simulink model "Quad_Cascade_PID"  (R2021b)
settings: Solver=ode45  StartTime=0.0  StopTime=t_sim  MaxStep=0.01  RelTol=1e-3  AbsTol=1e-6
values from neighbouring files (symbols this model uses):
  att_cmd_limit = 18 * pi/180    (= 0.314159265359)    [Quad_Params.m]
  AW_Phi = 0.5    [Quad_Params.m]
  AW_Psi = 0.3    [Quad_Params.m]
  AW_Theta = 0.5    [Quad_Params.m]
  AW_X = 0.5    [Quad_Params.m]
  AW_Y = 0.5    [Quad_Params.m]
  AW_Z = 3.0    (= 3)    [Quad_Params.m]
  B_torque = 0.0382    [Quad_Params.m]
  FF_X = 0.35    [Quad_Params.m]
  FF_Y = 0.40    (= 0.4)    [Quad_Params.m]
  g = 9.81    [Quad_Params.m]
  IXX = 4.856e-3    (= 0.004856)    [Quad_Params.m]
  IYY = 4.856e-3    (= 0.004856)    [Quad_Params.m]
  IZZ = 8.801e-3    (= 0.008801)    [Quad_Params.m]
  K_thrust = 2.98e-6    (= 2.98e-06)    [Quad_Params.m]
  KD_P = 0.010    (= 0.01)    [Quad_Params.m]
  KD_Phi = 0.80    (= 0.8)    [Quad_Params.m]
  KD_Psi = 0.40    (= 0.4)    [Quad_Params.m]
  KD_Q = 0.010    (= 0.01)    [Quad_Params.m]
  KD_R = 0.008    [Quad_Params.m]
  KD_Theta = 0.80    (= 0.8)    [Quad_Params.m]
  KD_X = 0.50    (= 0.5)    [Quad_Params.m]
  KD_Y = 0.70    (= 0.7)    [Quad_Params.m]
  KD_Z = 1.50    (= 1.5)    [Quad_Params.m]
  KI_P = 0.0001    [Quad_Params.m]
  KI_Phi = 0.0001    [Quad_Params.m]
  KI_Psi = 0.5    [Quad_Params.m]
  KI_Q = 0.0001    [Quad_Params.m]
  KI_R = 0.0001    [Quad_Params.m]
  KI_Theta = 0.0001    [Quad_Params.m]
  KI_X = 0.00    (= 0)    [Quad_Params.m]
  KI_Y = 0.00    (= 0)    [Quad_Params.m]
  KI_Z = 10.0    (= 10)    [Quad_Params.m]
  KP_P = 0.80    (= 0.8)    [Quad_Params.m]
  KP_Phi = 6.0    (= 6)    [Quad_Params.m]
  KP_Psi = 4.0    (= 4)    [Quad_Params.m]
  KP_Q = 0.80    (= 0.8)    [Quad_Params.m]
  KP_R = 0.60    (= 0.6)    [Quad_Params.m]
  KP_Theta = 6.0    (= 6)    [Quad_Params.m]
  KP_X = 0.80    (= 0.8)    [Quad_Params.m]
  KP_Y = 1.00    (= 1)    [Quad_Params.m]
  KP_Z = 10.0    (= 10)    [Quad_Params.m]
  L = 0.225    [Quad_Params.m]
  m = 0.468    [Quad_Params.m]    (also in quad_plant_fcn.m)
  M_max = L * K_thrust * omega_max^2    (= 0.6705)    [Quad_Params.m]
  N_rate = 50    [Quad_Params.m]
  omega_sq_max = omega_max^2    (= 1000000)    [Quad_Params.m]
  omega_sq_min = 0    [Quad_Params.m]
  Psid = 0.0    (= 0)    [Quad_Params.m]
  T_max = 4 * K_thrust * omega_max^2    (= 11.92)    [Quad_Params.m]
  T_min = 0    [Quad_Params.m]
  Ts_inner = 0.005    [Quad_Params.m]
  Ts_mid = 0.010    (= 0.01)    [Quad_Params.m]
  Ts_outer = 0.020    (= 0.02)    [Quad_Params.m]
  yaw_rate_limit = 1.0    (= 1)    [Quad_Params.m]
settings Model: Creator=ADMIN  LastModifiedBy=ADMIN
settings DataIOCC: SaveFormat=Array  ReturnWorkspaceOutputs=off

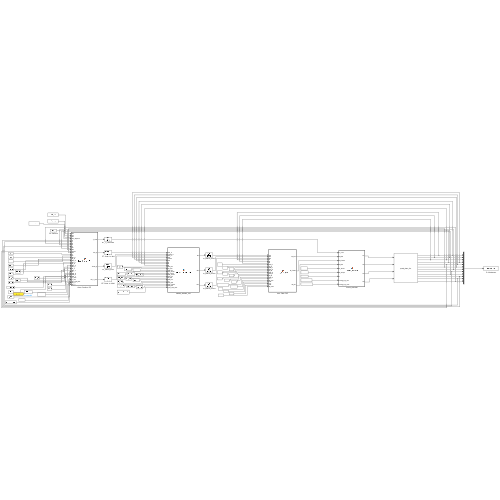
[thumbnail: Simulink's stored preview of the top-level diagram]
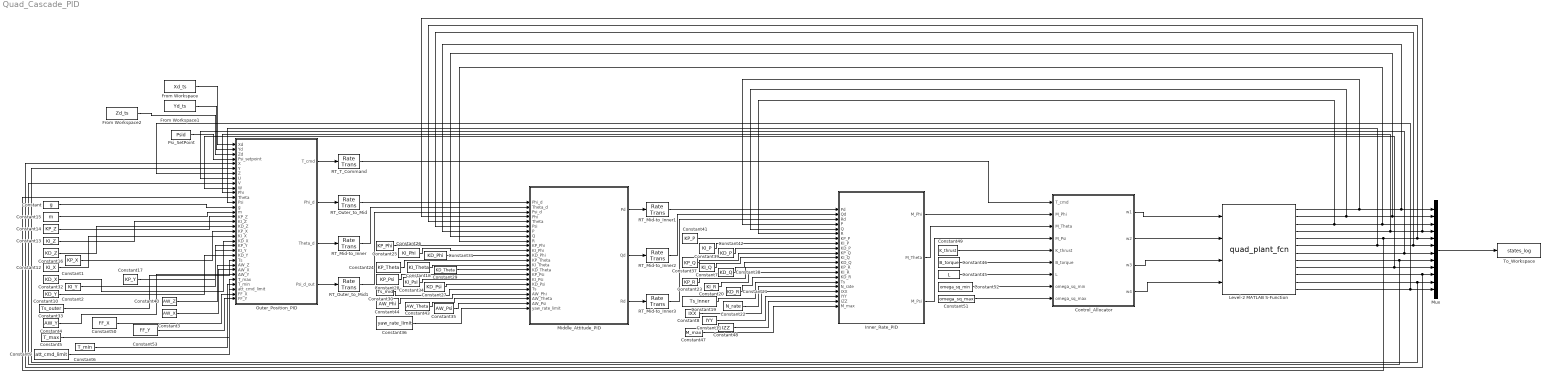
== system Quad_Cascade_PID ==
  Constant : Constant  Value=g
  Constant1 : Constant  Value=KP_X
  Constant10 : Constant  Value=KD_Y
  Constant11 : Constant  Value=IYY
  Constant12 : Constant  Value=KI_X
  Constant13 : Constant  Value=KI_Z
  Constant14 : Constant  Value=KP_Z
  Constant15 : Constant  Value=m
  Constant16 : Constant  Value=KD_Z
  Constant17 : Constant  Value=KP_Y
  Constant18 : Constant  Value=KI_Theta
  Constant19 : Constant  Value=Ts_inner
  Constant2 : Constant  Value=KI_Y
  Constant20 : Constant  Value=KI_R
  Constant21 : Constant  Value=KD_R
  Constant22 : Constant  Value=N_rate
  Constant23 : Constant  Value=KP_R
  Constant24 : Constant  Value=KP_Theta
  Constant25 : Constant  Value=KP_Phi
  Constant26 : Constant  Value=KI_Phi
  Constant27 : Constant  Value=KD_Psi
  Constant28 : Constant  Value=KP_Psi
  Constant29 : Constant  Value=KD_Theta
  Constant3 : Constant  Value=AW_X
  Constant30 : Constant  Value=Ts_mid
  Constant31 : Constant  Value=KD_Phi
  Constant32 : Constant  Value=KD_X
  Constant33 : Constant  Value=Ts_outer
  Constant34 : Constant  Value=KI_Psi
  Constant35 : Constant  Value=AW_Psi
  Constant36 : Constant  Value=yaw_rate_limit
  Constant37 : Constant  Value=KP_Q
  Constant38 : Constant  Value=KD_Q
  Constant39 : Constant  Value=KI_P
  Constant4 : Constant  Value=AW_Y
  Constant40 : Constant  Value=AW_Z
  Constant41 : Constant  Value=KP_P
  Constant42 : Constant  Value=KD_P
  Constant43 : Constant  Value=AW_Theta
  Constant44 : Constant  Value=AW_Phi
  Constant45 : Constant  Value=L
  Constant46 : Constant  Value=B_torque
  Constant47 : Constant  Value=M_max
  Constant48 : Constant  Value=IZZ
  Constant49 : Constant  Value=K_thrust
  Constant5 : Constant  Value=T_max
  Constant50 : Constant  Value=FF_X
  Constant51 : Constant  Value=omega_sq_max
  Constant52 : Constant  Value=omega_sq_min
  Constant53 : Constant  Value=FF_Y
  Constant6 : Constant  Value=T_min
  Constant7 : Constant  Value=KI_Q
  Constant8 : Constant  Value=IXX
  Constant9 : Constant  Value=att_cmd_limit
  Control_Allocator : MATLAB Function  TreatAsAtomicUnit=on
  From Workspace : FromWorkspace  VariableName=Xd_ts
  From Workspace1 : FromWorkspace  VariableName=Yd_ts
  From Workspace2 : FromWorkspace  VariableName=Zd_ts
  Inner_Rate_PID : MATLAB Function  TreatAsAtomicUnit=on  SystemSampleTime=Ts_inner
  Level-2 MATLAB S-Function : M-S-Function  FunctionName=quad_plant_fcn
  Middle_Attitude_PID : MATLAB Function  TreatAsAtomicUnit=on  SystemSampleTime=Ts_mid
  Mux : Mux  Inputs=12
  Outer_Position_PID : MATLAB Function  TreatAsAtomicUnit=on  SystemSampleTime=Ts_outer
  Psi_SetPoint : Constant  Value=Psid
  RT_Mid-to_Inner{,1..3} (4 alike) : RateTransition  Deterministic=off  OutPortSampleTime=Ts_inner
  RT_Outer_to_Mid : RateTransition  Deterministic=off  OutPortSampleTime=Ts_inner
  RT_Outer_to_Mid1 : RateTransition  Deterministic=off  OutPortSampleTime=Ts_inner
  RT_T_Command : RateTransition  Deterministic=off  OutPortSampleTime=Ts_inner
  To_Workspace : ToWorkspace  VariableName=states_log  SampleTime=-1
  wires:
  Level-2 MATLAB S-Function/1 -> Inner_Rate_PID/4(P), Middle_Attitude_PID/7(P), Mux/1
  Level-2 MATLAB S-Function/2 -> Inner_Rate_PID/5(Q), Middle_Attitude_PID/8(Q), Mux/2
  Level-2 MATLAB S-Function/3 -> Inner_Rate_PID/6(R), Middle_Attitude_PID/9(R), Mux/3
  Level-2 MATLAB S-Function/4 -> Middle_Attitude_PID/4(Phi), Mux/4, Outer_Position_PID/11(Phi)
  Level-2 MATLAB S-Function/5 -> Middle_Attitude_PID/5(Theta), Mux/5, Outer_Position_PID/12(Theta)
  Level-2 MATLAB S-Function/6 -> Middle_Attitude_PID/6(Psi), Mux/6, Outer_Position_PID/13(Psi)
  Level-2 MATLAB S-Function/7 -> Outer_Position_PID/8(U), Mux/7
  Level-2 MATLAB S-Function/8 -> Outer_Position_PID/9(V), Mux/8
  Level-2 MATLAB S-Function/9 -> Outer_Position_PID/10(W), Mux/9
  Level-2 MATLAB S-Function/10 -> Outer_Position_PID/5(X), Mux/10
  Level-2 MATLAB S-Function/11 -> Outer_Position_PID/6(Y), Mux/11
  Level-2 MATLAB S-Function/12 -> Outer_Position_PID/7(Z), Mux/12
  Mux/1 -> To_Workspace/1
  Psi_SetPoint/1 -> Outer_Position_PID/4(Psi_setpoint)
  Constant9/1 -> Outer_Position_PID/31(att_cmd_limit)
  Constant6/1 -> Outer_Position_PID/30(T_min)
  Constant5/1 -> Outer_Position_PID/29(T_max)
  Constant4/1 -> Outer_Position_PID/28(AW_Y)
  Constant3/1 -> Outer_Position_PID/27(AW_X)
  Constant40/1 -> Outer_Position_PID/26(AW_Z)
  Constant33/1 -> Outer_Position_PID/25(Ts)
  Constant10/1 -> Outer_Position_PID/24(KD_Y)
  Constant2/1 -> Outer_Position_PID/23(KI_Y)
  Constant17/1 -> Outer_Position_PID/22(KP_Y)
  Constant32/1 -> Outer_Position_PID/21(KD_X)
  Constant12/1 -> Outer_Position_PID/20(KI_X)
  Constant1/1 -> Outer_Position_PID/19(KP_X)
  Constant16/1 -> Outer_Position_PID/18(KD_Z)
  Constant13/1 -> Outer_Position_PID/17(KI_Z)
  Constant14/1 -> Outer_Position_PID/16(KP_Z)
  Constant15/1 -> Outer_Position_PID/15(m)
  Constant/1 -> Outer_Position_PID/14(g)
  Outer_Position_PID/1(T_cmd) -> RT_T_Command/1
  Outer_Position_PID/2(Phi_d) -> RT_Outer_to_Mid/1
  Outer_Position_PID/3(Theta_d) -> RT_Mid-to_Inner/1
  Outer_Position_PID/4(Psi_d_out) -> RT_Outer_to_Mid1/1
  RT_Outer_to_Mid/1 -> Middle_Attitude_PID/1(Phi_d)
  RT_Mid-to_Inner/1 -> Middle_Attitude_PID/2(Theta_d)
  RT_Outer_to_Mid1/1 -> Middle_Attitude_PID/3(Psi_d)
  Constant25/1 -> Middle_Attitude_PID/10(KP_Phi)
  Constant26/1 -> Middle_Attitude_PID/11(KI_Phi)
  Constant31/1 -> Middle_Attitude_PID/12(KD_Phi)
  Constant24/1 -> Middle_Attitude_PID/13(KP_Theta)
  Constant18/1 -> Middle_Attitude_PID/14(KI_Theta)
  Constant29/1 -> Middle_Attitude_PID/15(KD_Theta)
  Constant28/1 -> Middle_Attitude_PID/16(KP_Psi)
  Constant34/1 -> Middle_Attitude_PID/17(KI_Psi)
  Constant27/1 -> Middle_Attitude_PID/18(KD_Psi)
  Constant30/1 -> Middle_Attitude_PID/19(Ts)
  Constant44/1 -> Middle_Attitude_PID/20(AW_Phi)
  Constant43/1 -> Middle_Attitude_PID/21(AW_Theta)
  Constant35/1 -> Middle_Attitude_PID/22(AW_Psi)
  Constant36/1 -> Middle_Attitude_PID/23(yaw_rate_limit)
  Middle_Attitude_PID/1(Pd) -> RT_Mid-to_Inner1/1
  Middle_Attitude_PID/2(Qd) -> RT_Mid-to_Inner2/1
  Middle_Attitude_PID/3(Rd) -> RT_Mid-to_Inner3/1
  RT_Mid-to_Inner1/1 -> Inner_Rate_PID/1(Pd)
  RT_Mid-to_Inner2/1 -> Inner_Rate_PID/2(Qd)
  RT_Mid-to_Inner3/1 -> Inner_Rate_PID/3(Rd)
  Constant41/1 -> Inner_Rate_PID/7(KP_P)
  Constant39/1 -> Inner_Rate_PID/8(KI_P)
  Constant42/1 -> Inner_Rate_PID/9(KD_P)
  Constant37/1 -> Inner_Rate_PID/10(KP_Q)
  Constant7/1 -> Inner_Rate_PID/11(KI_Q)
  Constant38/1 -> Inner_Rate_PID/12(KD_Q)
  Constant23/1 -> Inner_Rate_PID/13(KP_R)
  Constant20/1 -> Inner_Rate_PID/14(KI_R)
  Constant21/1 -> Inner_Rate_PID/15(KD_R)
  Constant19/1 -> Inner_Rate_PID/16(Ts)
  Constant22/1 -> Inner_Rate_PID/17(N_rate)
  Constant8/1 -> Inner_Rate_PID/18(IXX)
  Constant11/1 -> Inner_Rate_PID/19(IYY)
  Constant48/1 -> Inner_Rate_PID/20(IZZ)
  Constant47/1 -> Inner_Rate_PID/21(M_max)
  Inner_Rate_PID/1(M_Phi) -> Control_Allocator/2(M_Phi)
  Inner_Rate_PID/2(M_Theta) -> Control_Allocator/3(M_Theta)
  Inner_Rate_PID/3(M_Psi) -> Control_Allocator/4(M_Psi)
  RT_T_Command/1 -> Control_Allocator/1(T_cmd)
  Constant49/1 -> Control_Allocator/5(K_thrust)
  Constant46/1 -> Control_Allocator/6(B_torque)
  Constant45/1 -> Control_Allocator/7(L)
  Constant52/1 -> Control_Allocator/8(omega_sq_min)
  Constant51/1 -> Control_Allocator/9(omega_sq_max)
  Control_Allocator/1(w1) -> Level-2 MATLAB S-Function/1
  Control_Allocator/2(w2) -> Level-2 MATLAB S-Function/2
  Control_Allocator/3(w3) -> Level-2 MATLAB S-Function/3
  Control_Allocator/4(w4) -> Level-2 MATLAB S-Function/4
  From Workspace2/1 -> Outer_Position_PID/3(Zd)
  From Workspace1/1 -> Outer_Position_PID/2(Yd)
  From Workspace/1 -> Outer_Position_PID/1(Xd)
  Constant50/1 -> Outer_Position_PID/32(FF_X)
  Constant53/1 -> Outer_Position_PID/33(FF_Y)

== matlab function Quad_Cascade_PID/Inner_Rate_PID ==
  data: Pd input; M_Phi output; Qd input; Rd input; P input; Q input; R input; M_Theta output; M_Psi output; KP_P input; KI_P input; KD_P input; KP_Q input; KI_Q input; KD_Q input; KP_R input; KI_R input; KD_R input; Ts input; N_rate input; IXX input; IYY input; IZZ input; M_max input
function [M_Phi, M_Theta, M_Psi] = Inner_Rate_PID(...
    Pd, Qd, Rd, P, Q, R, ...
    KP_P, KI_P, KD_P, ...
    KP_Q, KI_Q, KD_Q, ...
    KP_R, KI_R, KD_R, ...
    Ts, N_rate, ...
    IXX, IYY, IZZ, M_max)

% INNER RATE PID
% All parameters passed directly as input ports

% Persistent states
persistent int_P int_Q int_R prev_eP prev_eQ prev_eR first_run

if isempty(first_run)
    int_P    = 0;   int_Q    = 0;   int_R    = 0;
    prev_eP  = 0;   prev_eQ  = 0;   prev_eR  = 0;
    first_run = false;
end

% =============================================
% RATE ERRORS
% =============================================

eP = Pd - P;
eQ = Qd - Q;
eR = Rd - R;

% =============================================
% INTEGRATOR UPDATE (Tustin)
% =============================================

int_P = int_P + (Ts/2) * (eP + prev_eP);
int_Q = int_Q + (Ts/2) * (eQ + prev_eQ);
int_R = int_R + (Ts/2) * (eR + prev_eR);

% =============================================
% DERIVATIVE WITH FILTER
% =============================================

dP = N_rate * (eP - prev_eP) / (1 + N_rate * Ts);
dQ = N_rate * (eQ - prev_eQ) / (1 + N_rate * Ts);
dR = N_rate * (eR - prev_eR) / (1 + N_rate * Ts);

% =============================================
% PID OUTPUT — torque commands
% Multiply by inertia for physical units [N.m]
% =============================================

M_Phi_raw   = IXX * (KP_P * eP + KI_P * int_P + KD_P * dP);
M_Theta_raw = IYY * (KP_Q * eQ + KI_Q * int_Q + KD_Q * dQ);
M_Psi_raw   = IZZ * (KP_R * eR + KI_R * int_R + KD_R * dR);

% Saturate torques
M_Phi   = max(-M_max, min(M_max, M_Phi_raw));
M_Theta = max(-M_max, min(M_max, M_Theta_raw));
M_Psi   = max(-M_max, min(M_max, M_Psi_raw));

% Back-calculation anti-windup
AW_gain = 0.1;
int_P = int_P + AW_gain * (M_Phi   - M_Phi_raw)   / (IXX * KI_P + eps);
int_Q = int_Q + AW_gain * (M_Theta - M_Theta_raw) / (IYY * KI_Q + eps);
int_R = int_R + AW_gain * (M_Psi   - M_Psi_raw)   / (IZZ * KI_R + eps);

% =============================================
% UPDATE MEMORY
% =============================================

prev_eP = eP;
prev_eQ = eQ;
prev_eR = eR;

end

== matlab function Quad_Cascade_PID/Control_Allocator ==
  data: T_cmd input; w1 output; M_Phi input; M_Theta input; M_Psi input; w2 output; w3 output; w4 output; K_thrust input; B_torque input; L input; omega_sq_min input; omega_sq_max input
function [w1, w2, w3, w4] = Control_Allocator(...
    T_cmd, M_Phi, M_Theta, M_Psi, ...
    K_thrust, B_torque, L, ...
    omega_sq_min, omega_sq_max)

% CONTROL ALLOCATOR
% All parameters passed directly as input ports

% =============================================
% STEP 1: Compute omega squared (Eq. 3.24)
% =============================================

T_over_4K      = T_cmd    / (4 * K_thrust);
M_theta_term   = M_Theta  / (2 * K_thrust * L);
M_phi_term     = M_Phi    / (2 * K_thrust * L);
M_psi_term     = M_Psi    / (4 * B_torque);

w1_sq = T_over_4K - M_theta_term - M_psi_term;
w2_sq = T_over_4K - M_phi_term   + M_psi_term;
w3_sq = T_over_4K + M_theta_term - M_psi_term;
w4_sq = T_over_4K + M_phi_term   + M_psi_term;

% =============================================
% STEP 2: Physical saturation
% omega squared cannot be negative
% =============================================

w1_sq = max(omega_sq_min, min(omega_sq_max, w1_sq));
w2_sq = max(omega_sq_min, min(omega_sq_max, w2_sq));
w3_sq = max(omega_sq_min, min(omega_sq_max, w3_sq));
w4_sq = max(omega_sq_min, min(omega_sq_max, w4_sq));

% =============================================
% STEP 3: Square root to get rotor speeds
% =============================================

w1 = sqrt(w1_sq);
w2 = sqrt(w2_sq);
w3 = sqrt(w3_sq);
w4 = sqrt(w4_sq);

end

== matlab function Quad_Cascade_PID/Middle_Attitude_PID ==
  data: Phi_d input; Pd output; Theta_d input; Psi_d input; Phi input; Theta input; Psi input; P input; Q input; R input; Qd output; Rd output; KP_Phi input; KI_Phi input; KD_Phi input; KP_Theta input; KI_Theta input; KD_Theta input; KP_Psi input; KI_Psi input; KD_Psi input; Ts input; AW_Phi input; AW_Theta input; AW_Psi input; yaw_rate_limit input
function [Pd, Qd, Rd] = Middle_Attitude_PID(...
    Phi_d, Theta_d, Psi_d, ...
    Phi, Theta, Psi, P, Q, R, ...
    KP_Phi, KI_Phi, KD_Phi, ...
    KP_Theta, KI_Theta, KD_Theta, ...
    KP_Psi, KI_Psi, KD_Psi, ...
    Ts, AW_Phi, AW_Theta, AW_Psi, ...
    yaw_rate_limit)

% MIDDLE ATTITUDE PID
% All parameters passed directly as input ports

% Persistent integrator states
persistent int_Phi int_Theta int_Psi first_run

if isempty(first_run)
    int_Phi   = 0;
    int_Theta = 0;
    int_Psi   = 0;
    first_run = false;
end

% =============================================
% ANGLE ERRORS
% =============================================

e_Phi   = Phi_d   - Phi;
e_Theta = Theta_d - Theta;

% Wrap yaw error to [-pi, pi]
e_Psi_raw = Psi_d - Psi;
e_Psi     = atan2(sin(e_Psi_raw), cos(e_Psi_raw));

% =============================================
% INTEGRATOR UPDATE
% =============================================

int_Phi   = int_Phi   + Ts * e_Phi;
int_Theta = int_Theta + Ts * e_Theta;
int_Psi   = int_Psi   + Ts * e_Psi;

% Anti-windup clamping
int_Phi   = max(-AW_Phi/KI_Phi,     min(AW_Phi/KI_Phi,     int_Phi));
int_Theta = max(-AW_Theta/KI_Theta, min(AW_Theta/KI_Theta, int_Theta));
int_Psi   = max(-AW_Psi/KI_Psi,     min(AW_Psi/KI_Psi,     int_Psi));

% =============================================
% DERIVATIVE ON MEASUREMENT
% Uses actual rates P, Q, R instead of
% differentiating error — no derivative kick
% =============================================

dPhi_meas   = -P;
dTheta_meas = -Q;
dPsi_meas   = -R;

% =============================================
% PID OUTPUT — desired angular rates
% =============================================

rate_lim = yaw_rate_limit * 3;

Pd_raw = KP_Phi   * e_Phi   + KI_Phi   * int_Phi   + KD_Phi   * dPhi_meas;
Qd_raw = KP_Theta * e_Theta + KI_Theta * int_Theta + KD_Theta * dTheta_meas;
Rd_raw = KP_Psi   * e_Psi   + KI_Psi   * int_Psi   + KD_Psi   * dPsi_meas;

% Saturate output rates
Pd = max(-rate_lim,        min(rate_lim,        Pd_raw));
Qd = max(-rate_lim,        min(rate_lim,        Qd_raw));
Rd = max(-yaw_rate_limit,  min(yaw_rate_limit,  Rd_raw));

end

== matlab function Quad_Cascade_PID/Outer_Position_PID ==
  data: Xd input; T_cmd output; Yd input; Zd input; Psi_setpoint input; X input; Y input; Z input; U input; V input; W input; Phi input; Theta input; Psi input; Phi_d output; Theta_d output; Psi_d_out output; g input; m input; KP_Z input; KI_Z input; KD_Z input; KP_X input; KI_X input; KD_X input; KP_Y input; KI_Y input; KD_Y input; Ts input; AW_Z input; AW_X input; AW_Y input; T_max input; T_min input; att_cmd_limit input; FF_X input; FF_Y input
function [T_cmd, Phi_d, Theta_d, Psi_d_out] = Outer_Position_PID(...
    Xd, Yd, Zd, Psi_setpoint, ...
    X, Y, Z, U, V, W, Phi, Theta, Psi, ...
    g, m, ...
    KP_Z, KI_Z, KD_Z, ...
    KP_X, KI_X, KD_X, ...
    KP_Y, KI_Y, KD_Y, ...
    Ts, AW_Z, AW_X, AW_Y, ...
    T_max, T_min, att_cmd_limit, ...
    FF_X, FF_Y)

% OUTER POSITION PID
% All parameters passed directly as input ports
% FF_X and FF_Y are feedforward gains for X and Y axes

% Persistent integrator states
persistent int_Z int_X int_Y first_run Xd_prev Yd_prev

if isempty(first_run)
    int_Z     = 0;
    int_X     = 0;
    int_Y     = 0;
    Xd_prev   = Xd;
    Yd_prev   = Yd;
    first_run = false;
end

% =============================================
% ALTITUDE CONTROLLER (Z axis)
% =============================================

e_Z = Zd - Z;

% Integrator update
int_Z = int_Z + Ts * e_Z;

% Anti-windup clamping
int_Z = max(-AW_Z, min(AW_Z, int_Z));

% Derivative on measurement
dZ_meas = -W;

% PID output
az_cmd = KP_Z * e_Z + KI_Z * int_Z + KD_Z * dZ_meas;

% Thrust command with gravity feedforward
cos_corr = cos(Phi) * cos(Theta);
cos_corr = max(0.5, cos_corr);
T_raw    = m * (g + az_cmd) / cos_corr;

% Saturate thrust
T_cmd = max(T_min, min(T_max, T_raw));

% =============================================
% HORIZONTAL POSITION CONTROLLER (X, Y)
% =============================================

% Inertial position errors
e_X_inertial = Xd - X;
e_Y_inertial = Yd - Y;

% Rotate to body frame using current yaw
e_X_body =  e_X_inertial * cos(Psi) + e_Y_inertial * sin(Psi);
e_Y_body =  e_Y_inertial * cos(Psi) - e_X_inertial * sin(Psi);

% Desired body velocities
Ud_desired = e_X_body;
Vd_desired = e_Y_body;

% Velocity errors
e_U = Ud_desired - U;
e_V = Vd_desired - V;

% Integrator update with anti-windup
int_X = int_X + Ts * e_U;
int_Y = int_Y + Ts * e_V;
int_X = max(-AW_X, min(AW_X, int_X));
int_Y = max(-AW_Y, min(AW_Y, int_Y));

% Derivative on measurement
dU_meas = -U;
dV_meas = -V;

% =============================================
% FEEDFORWARD CALCULATION
%
% PURPOSE:
%   Normal PID reacts AFTER error builds up.
%   Feedforward predicts where reference is going
%   and acts BEFORE error builds up.
%   This reduces phase lag between lime green and yellow paths.
%
% METHOD:
%   Finite difference of Xd and Yd gives reference velocity.
%   Xd_dot = (Xd_now - Xd_previous) / Ts
%   Yd_dot = (Yd_now - Yd_previous) / Ts
%   Velocity is rotated to body frame using Psi.
%   Then added directly to PID attitude output.
%
% TUNING:
%   FF_X = FF_Y = 0.0  → no feedforward (pure PID)
%   FF_X = FF_Y = 0.5  → medium (current setting)
%   FF_X = FF_Y = 1.0  → strong
%   Cyan lags behind yellow  → increase FF_X, FF_Y
%   Cyan overshoots yellow   → decrease FF_X, FF_Y
% =============================================

% Reference velocity using finite difference
Xd_dot_ref = (Xd - Xd_prev) / Ts;
Yd_dot_ref = (Yd - Yd_prev) / Ts;

% Update memory for next step
Xd_prev = Xd;
Yd_prev = Yd;

% Rotate reference velocity from inertial to body frame
Xd_dot_body =  Xd_dot_ref * cos(Psi) + Yd_dot_ref * sin(Psi);
Yd_dot_body =  Yd_dot_ref * cos(Psi) - Xd_dot_ref * sin(Psi);

% Feedforward attitude commands
ff_theta =  FF_X * Xd_dot_body;
ff_phi   = -FF_Y * Yd_dot_body;

% =============================================
% PID + FEEDFORWARD COMBINED OUTPUT
% =============================================

Theta_d_raw =  (KP_X * e_U + KI_X * int_X + KD_X * dU_meas) + ff_theta;
Phi_d_raw   = -(KP_Y * e_V + KI_Y * int_Y + KD_Y * dV_meas) + ff_phi;

% Saturate attitude commands
Theta_d   = max(-att_cmd_limit, min(att_cmd_limit, Theta_d_raw));
Phi_d     = max(-att_cmd_limit, min(att_cmd_limit, Phi_d_raw));

% Pass through yaw setpoint
Psi_d_out = Psi_setpoint;

end
